simulink model "Red_problema6_rndm"  (R2021a)
settings: Solver=ode15s  StartTime=0.0  StopTime=sim_time  RelTol=1e-3
values from neighbouring files (symbols this model uses):
  aE112 = 177.25533427288616    (= 177.255334273)    [data_run_lazo_abierto_simulink.m]    (also in inicializar_areas.m = 179.376259805; script_IMC.m = a112_f)
  aE121 = 28.272251308900536    (= 28.2722513089)    [data_run_lazo_abierto_simulink.m]    (also in inicializar_areas.m; script_IMC.m = a121_f)
  aE213 = 304.960661680865    (= 304.960661681)    [data_run_lazo_abierto_simulink.m]    (also in inicializar_areas.m; script_IMC.m = a213_f)
  aE222 = 104.78323167686085    (= 104.783231677)    [data_run_lazo_abierto_simulink.m]    (also in inicializar_areas.m = 114.075570199; script_IMC.m = a222_f)
  aEcu1 = 2.44278466343862    (= 2.44278466344)    [data_run_lazo_abierto_simulink.m]    (also in inicializar_areas.m = 4.955447053)
  aEcu2 = 9.34130944614368    (= 9.34130944614)    [data_run_lazo_abierto_simulink.m]    (also in inicializar_areas.m = 18.78773145)
  aEhu2 = 53.1053199018638    (= 53.1053199019)    [data_run_lazo_abierto_simulink.m]    (also in inicializar_areas.m = 53.1053199)
  d1_end = 0    [data_run_lazo_abierto_simulink.m]    (also in inicializar_entradas.m; pert_max.m = 0.99; script_build_tfs.m)
  d1_in = 0    [data_run_lazo_abierto_simulink.m]    (also in inicializar_entradas.m; script_build_tfs.m)
  d2_end = 0    [data_run_lazo_abierto_simulink.m]    (also in inicializar_entradas.m; pert_max.m = 0.15; script_build_tfs.m)
  d2_in = 0    [data_run_lazo_abierto_simulink.m]    (also in inicializar_entradas.m; script_build_tfs.m)
  d3_end = 0    [data_run_lazo_abierto_simulink.m]    (also in inicializar_entradas.m; pert_max.m = 0.99; script_build_tfs.m)
  d3_in = 0    [data_run_lazo_abierto_simulink.m]    (also in inicializar_entradas.m; script_build_tfs.m)
  d4_end = 0    [data_run_lazo_abierto_simulink.m]    (also in inicializar_entradas.m; pert_max.m = 0.15; script_build_tfs.m)
  d4_in = 0    [data_run_lazo_abierto_simulink.m]    (also in inicializar_entradas.m; script_build_tfs.m)
  d5_end = 0    [data_run_lazo_abierto_simulink.m]    (also in inicializar_entradas.m; pert_max.m = -0.99; script_build_tfs.m)
  d5_in = 0    [data_run_lazo_abierto_simulink.m]    (also in inicializar_entradas.m; script_build_tfs.m)
  d6_end = 0    [data_run_lazo_abierto_simulink.m]    (also in inicializar_entradas.m; pert_max.m = 0.15; script_build_tfs.m)
  d6_in = 0    [data_run_lazo_abierto_simulink.m]    (also in inicializar_entradas.m; script_build_tfs.m)
  d7_end = 0    [data_run_lazo_abierto_simulink.m]    (also in inicializar_entradas.m; pert_max.m = -0.99; script_build_tfs.m)
  d7_in = 0    [data_run_lazo_abierto_simulink.m]    (also in inicializar_entradas.m; script_build_tfs.m)
  d8_end = 0    [data_run_lazo_abierto_simulink.m]    (also in inicializar_entradas.m; pert_max.m = 0.15; script_build_tfs.m)
  d8_in = 0    [data_run_lazo_abierto_simulink.m]    (also in inicializar_entradas.m; script_build_tfs.m)
  est = 1    [data_run_lazo_abierto_simulink.m]    (also in ini_comun.m; script_build_tfs.m)
  fc1 = 20    [data_run_lazo_abierto_simulink.m]    (also in ini_comun.m; script_build_tfs.m)
  fc2 = 50    [data_run_lazo_abierto_simulink.m]    (also in ini_comun.m; script_build_tfs.m)
  fcu1 = 36    [data_run_lazo_abierto_simulink.m]    (also in ini_comun.m = 1.45; inicializar_areas.m = 1.45; script_build_tfs.m = 1.45)
  fcu2 = 44    [data_run_lazo_abierto_simulink.m]    (also in ini_comun.m = 5; inicializar_areas.m = 5; script_build_tfs.m = 5)
  fh1 = 18    [data_run_lazo_abierto_simulink.m]    (also in ini_comun.m; script_build_tfs.m)
  fh2 = 22    [data_run_lazo_abierto_simulink.m]    (also in ini_comun.m; script_build_tfs.m)
  fhu2 = 14.8    [data_run_lazo_abierto_simulink.m]    (also in ini_comun.m = 15; inicializar_areas.m = 15; script_build_tfs.m = 15)
  hc1 = 1    [data_run_lazo_abierto_simulink.m]    (also in ini_comun.m; script_build_tfs.m)
  hc2 = 1    [data_run_lazo_abierto_simulink.m]    (also in ini_comun.m; script_build_tfs.m)
  hcu = 1    [data_run_lazo_abierto_simulink.m]    (also in ini_comun.m; script_build_tfs.m)
  hh1 = 1    [data_run_lazo_abierto_simulink.m]    (also in ini_comun.m; script_build_tfs.m)
  hh2 = 1    [data_run_lazo_abierto_simulink.m]    (also in ini_comun.m; script_build_tfs.m)
  hhu = 1    [data_run_lazo_abierto_simulink.m]    (also in ini_comun.m; script_build_tfs.m)
  nom_ini = initials    [data_run_lazo_abierto_simulink.m]    (also in script_build_tfs.m)
  s1 = 30    [data_run_lazo_abierto_simulink.m]    (also in ini_comun.m; script_build_tfs.m)
  salida_pto_op = [432.97111685 332.893814589 483.000816221 482.974592221]    [D_desc_v1.mat]    (also in D_full_v1.mat = [432.946215914 332.89088523 483.00068651 483.133358057]; D_spar_v1.mat = [432.948244916 332.889043395 483.001208597 483.133835705]; G_modelo_desc_v2.mat = [432.971365599 332.894094109 483.00091452 482.974592221]; G_modelo_desc_v3.mat = [432.971116863 332.893814604 483.000816226 482.974592221])
  t_step = 2000    [data_run_lazo_abierto_simulink.m]    (also in ini_comun.m = 20000; script_build_tfs.m = 1000)
  Tcin1 = 323    [data_run_lazo_abierto_simulink.m]    (also in ini_comun.m; script_build_tfs.m)
  Tcin2 = 433    [data_run_lazo_abierto_simulink.m]    (also in ini_comun.m; script_build_tfs.m)
  Tcuin = 288    [data_run_lazo_abierto_simulink.m]    (also in ini_comun.m; script_build_tfs.m)
  Thin1 = 543    [data_run_lazo_abierto_simulink.m]    (also in ini_comun.m; script_build_tfs.m)
  Thin2 = 493    [data_run_lazo_abierto_simulink.m]    (also in ini_comun.m; script_build_tfs.m)
  Thuin = 523    [data_run_lazo_abierto_simulink.m]    (also in ini_comun.m; script_build_tfs.m)
  u10_end = nom_ini(10)    [data_run_lazo_abierto_simulink.m]    (also in inicializar_entradas.m = initials(10); script_build_tfs.m)
  u10_in = nom_ini(10)    [data_run_lazo_abierto_simulink.m]    (also in inicializar_entradas.m = initials(10); script_build_tfs.m)
  u11_end = nom_ini(11)    [data_run_lazo_abierto_simulink.m]    (also in inicializar_entradas.m = initials(11); script_build_tfs.m)
  u11_in = nom_ini(11)    [data_run_lazo_abierto_simulink.m]    (also in inicializar_entradas.m = initials(11); script_build_tfs.m)
  u1_end = nom_ini(1)    [data_run_lazo_abierto_simulink.m]    (also in inicializar_entradas.m = initials(1); script_build_tfs.m)
  u1_in = nom_ini(1)    [data_run_lazo_abierto_simulink.m]    (also in inicializar_entradas.m = initials(1); script_build_tfs.m)
  u2_end = nom_ini(2)    [data_run_lazo_abierto_simulink.m]    (also in inicializar_entradas.m = initials(2); script_build_tfs.m)
  u2_in = nom_ini(2)    [data_run_lazo_abierto_simulink.m]    (also in inicializar_entradas.m = initials(2); script_build_tfs.m)
  u3_end = nom_ini(3)    [data_run_lazo_abierto_simulink.m]    (also in inicializar_entradas.m = initials(3); script_build_tfs.m)
  u3_in = nom_ini(3)    [data_run_lazo_abierto_simulink.m]    (also in inicializar_entradas.m = initials(3); script_build_tfs.m)
  u4_end = nom_ini(4)    [data_run_lazo_abierto_simulink.m]    (also in inicializar_entradas.m = initials(4); script_build_tfs.m)
  u4_in = nom_ini(4)    [data_run_lazo_abierto_simulink.m]    (also in inicializar_entradas.m = initials(4); script_build_tfs.m)
  u5_end = nom_ini(5)    [data_run_lazo_abierto_simulink.m]    (also in inicializar_entradas.m = initials(5); script_build_tfs.m)
  u5_in = nom_ini(5)    [data_run_lazo_abierto_simulink.m]    (also in inicializar_entradas.m = initials(5); script_build_tfs.m)
  u6_end = nom_ini(6)    [data_run_lazo_abierto_simulink.m]    (also in inicializar_entradas.m = initials(6); script_build_tfs.m)
  u6_in = nom_ini(6)    [data_run_lazo_abierto_simulink.m]    (also in inicializar_entradas.m = initials(6); script_build_tfs.m)
  u7_end = nom_ini(7)    [data_run_lazo_abierto_simulink.m]    (also in inicializar_entradas.m = initials(7); script_build_tfs.m)
  u7_in = nom_ini(7)    [data_run_lazo_abierto_simulink.m]    (also in inicializar_entradas.m = initials(7); script_build_tfs.m)
  u8_end = nom_ini(8)    [data_run_lazo_abierto_simulink.m]    (also in inicializar_entradas.m = initials(8); script_build_tfs.m)
  u8_in = nom_ini(8)    [data_run_lazo_abierto_simulink.m]    (also in inicializar_entradas.m = initials(8); script_build_tfs.m)
  u9_end = nom_ini(9)    [data_run_lazo_abierto_simulink.m]    (also in inicializar_entradas.m = initials(9); script_build_tfs.m)
  u9_in = nom_ini(9)    [data_run_lazo_abierto_simulink.m]    (also in inicializar_entradas.m = initials(9); script_build_tfs.m)
undefined symbols (not defined in the file or in its folder): amp_time, bypass_time, fail_constant, interval_time
libraries: simulink x34, cstblocks x1
(part 1 of 2)
settings Model: Creator=Lautaro  LastModifiedBy=fzpat
settings SolverCC: AlgebraicLoopSolver=TrustRegion
settings DataIOCC: InitialState=xFinal  LimitDataPoints=on  SaveFinalState=on  SaveFormat=Array  ReturnWorkspaceOutputs=off
settings OptimizationCC: BlockReduction=off  BooleanDataType=off  LifeSpan=inf
settings DebuggingCC: SaveWithParameterizedLinksMsg=none  UnderspecifiedInitializationDetection=Classic  MergeDetectMultiDrivingBlocksExec=none  SignalResolutionControl=TryResolveAllWithWarning  SFUnexpectedBacktrackingDiag=warning  SFNoUnconditionalDefaultTransitionDiag=warning  SFExecutionAtInitializationDiag=none  SFMachineParentedDataDiag=warning  ArithmeticOperatorsInVariantConditions=warning
settings HardwareCC: ProdBitPerPointer=32  ProdBitPerSizeT=32  ProdBitPerPtrDiffT=32  ProdLargestAtomicFloat=None  ProdIntDivRoundTo=Undefined  ProdEndianess=Unspecified  ProdWordSize=32  ProdHWDeviceType=32-bit Generic  TargetUnknown=on
settings ModelReferenceCC: PropagateSignalLabelsOutOfModel=off
settings SFSimCC: SimUseLocalCustomCode=off  CustomCodeUndefinedFunction=UseInterfaceOnly
settings RTWCC: RTWUseLocalCustomCode=off
settings CodeAppCC: StateflowObjectComments=on
settings GRTTargetCC: TargetLangStandard=C89/C90 (ANSI)
settings ConfigComp: CovMetricSettings=dw  CovSaveCumulativeToWorkspaceVar=on  CovSaveSingleToWorkspaceVar=on  CovExternalEMLEnable=off  CovSFcnEnable=off

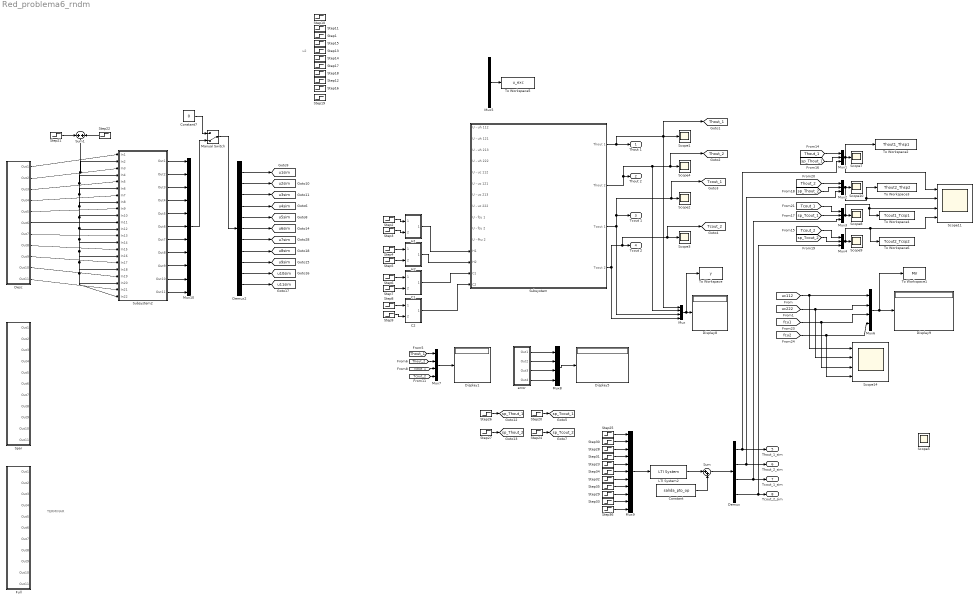
== system Red_problema6_rndm ==
  note: TERMINAR
  note: u2
  C1 : Subsystem
  "C2 " : Subsystem
  Constant : Constant  Value=salida_pto_op
  Constant7 : Constant  Value=0
  Demux : Demux
  Demux2 : Demux  Outputs=11
  Desc : Subsystem
  Display{1,5,8..9} (4 alike) : Display
  Full : Subsystem
  "H1 " : Subsystem
  H2 : Subsystem
  LTI System2 : cstblocks/LTI System  sys=G_modelo  IC=[]
  Manual Switch : ManualSwitch  CurrentSetting=0
  Mux{,6..8} (4 alike) : Mux
  Mux{1..4} (4 alike) : Mux  Inputs=3
  Mux10 : Mux  Inputs=11
  Mux5 : Mux  Inputs=11
  Mux9 : Mux  Inputs=11
  Scope{1..5,7..10} (9 alike) : Scope
  Scope11 : Scope  NumInputPorts=4
  Scope14 : Scope  NumInputPorts=4
  Spar : Subsystem
  Step1 : Step  Time=t_step  Before=u5_in  After=u5_end
  Step10 : Step  Time=t_step  Before=u1_in  After=u1_end
  Step11 : Step  Time=t_step  Before=u3_in  After=u3_end
  Step12 : Step  Time=t_step  Before=u9_in  After=u9_end
  Step13 : Step  Time=t_step  Before=u2_in  After=u2_end
  Step14 : Step  Time=t_step  Before=u4_in  After=u4_end
  Step15 : Step  Time=t_step  Before=u7_in  After=u7_end
  Step16 : Step  Time=t_step  Before=u10_in  After=u10_end
  Step17 : Step  Time=t_step  Before=u6_in  After=u6_end
  Step18 : Step  Time=t_step  Before=u8_in  After=u8_end
  Step19 : Step  Time=t_step  Before=u11_in  After=u11_end
  Step2 : Step  Time=t_step  Before=d1_in  After=d1_end
  Step20 : Step  Time=1e9  Before=210+273  After=210+273
  Step21 : Step  Time=bypass_time
  Step22 : Step  Time=bypass_time+125  After=-1
  Step23 : Step  Time=t_step  Before=u5_in - u5_in  After=u5_end - u5_in
  Step24 : Step  Time=1e10  Before=210+273  After=210+273
  Step25 : Step  Time=t_step  Before=u1_in - u1_in  After=u1_end - u1_in
  Step26 : Step  Time=1e9  Before=160+273  After=160+273
  Step27 : Step  Time=1e9  Before=60+273  After=60+273
  Step28 : Step  Time=t_step  Before=u3_in - u3_in  After=u3_end - u3_in
  Step29 : Step  Time=t_step  Before=u9_in - u9_in  After=u9_end - u9_in
  Step3 : Step  Time=t_step  Before=d2_in  After=d2_end
  Step30 : Step  Time=t_step  Before=u2_in - u2_in  After=u2_end - u2_in
  Step31 : Step  Time=t_step  Before=u4_in - u4_in  After=u4_end - u4_in
  Step32 : Step  Time=t_step  Before=u7_in - u7_in  After=u7_end - u7_in
  Step33 : Step  Time=t_step  Before=u10_in - u10_in  After=u10_end - u10_in
  Step34 : Step  Time=t_step  Before=u6_in - u6_in  After=u6_end - u6_in
  Step35 : Step  Time=t_step  Before=u8_in - u8_in  After=u8_end - u8_in
  Step36 : Step  Time=t_step  Before=u11_in - u11_in  After=u11_end - u11_in
  Step4 : Step  Time=t_step  Before=d3_in  After=d3_end
  Step5 : Step  Time=t_step  Before=d4_in  After=d4_end
  Step6 : Step  Time=t_step  Before=d5_in  After=d5_end
  Step7 : Step  Time=t_step  Before=d6_in  After=d6_end
  Step8 : Step  Time=t_step  Before=d7_in  After=d7_end
  Step9 : Step  Time=t_step  Before=d8_in  After=d8_end
  Subsystem : Subsystem
  Subsystem2 : Subsystem
  Sum : Sum  Inputs=|++
  Sum1 : Sum
  To Workspace : ToWorkspace  VariableName=y  SaveFormat=Timeseries  SampleTime=-1
  To Workspace1 : ToWorkspace  VariableName=MV  SaveFormat=Timeseries  SampleTime=-1
  To Workspace2 : ToWorkspace  VariableName=Thout1_Thsp1  SaveFormat=Timeseries  SampleTime=-1
  To Workspace3 : ToWorkspace  VariableName=Thout2_Thsp2  SampleTime=-1
  To Workspace4 : ToWorkspace  VariableName=Tcout1_Tcsp1  SampleTime=-1
  To Workspace5 : ToWorkspace  VariableName=u_exc  SaveFormat=Timeseries  SampleTime=-1
      settings: Save2DSignal=2-D array (concatenate along first dimension)
  To Workspace6 : ToWorkspace  VariableName=Tcout2_Tcsp2  SampleTime=-1
  error : Subsystem
  Thout 1 : Outport  VectorParamsAs1DForOutWhenUnconnected=off
  Thout 2 : Outport  Port=2  VectorParamsAs1DForOutWhenUnconnected=off
  Tcout 1 : Outport  Port=3  VectorParamsAs1DForOutWhenUnconnected=off
  Tcout 2 : Outport  Port=4  VectorParamsAs1DForOutWhenUnconnected=off
  Thout_1_sim : Outport  Port=5  VectorParamsAs1DForOutWhenUnconnected=off
  Thout_2_sim : Outport  Port=6  VectorParamsAs1DForOutWhenUnconnected=off
  Tcout_1_sim : Outport  Port=7  VectorParamsAs1DForOutWhenUnconnected=off
  Tcout_2_sim : Outport  Port=8  VectorParamsAs1DForOutWhenUnconnected=off
  tag scope: Tcout_1=global, Tcout_2=global, Thout_1=global, Thout_2=global, sp_Tcout_1=global, sp_Tcout_2=global, sp_Thout_1=global, sp_Thout_2=global, u10sim=global, u11sim=global, u1sim=global, u2sim=global, u3sim=global, u4sim=global, u5sim=global, u6sim=global, u7sim=global, u8sim=global, u9sim=global
  wires:
  Subsystem/1(Thout 1) -> Mux/1, Scope1/1, [Thout_1], Thout 1/1
  Mux/1 -> To Workspace/1, Display8/1
  "H1 "/1(Out1) -> Subsystem/12(H1)
  H2/1(Out1) -> Subsystem/13(H2)
  C1/1(Out1) -> Subsystem/14(C1)
  "C2 "/1(Out1) -> Subsystem/15(C2)
  Subsystem/2(Thout 2) -> [Thout_2], Scope4/1, Mux/2, Thout 2/1
  Subsystem/3(Tcout 1) -> [Tcout_1], Scope2/1, Tcout 1/1, Mux/3
  Step2/1 -> "H1 "/1(Thin 1)
  Step3/1 -> "H1 "/2(fhin 1)
  Step4/1 -> H2/1(Thin 2)
  Step5/1 -> H2/2(fhin 2)
  Step6/1 -> C1/1(Tcin 1)
  Step7/1 -> C1/2(fcin 1)
  Step8/1 -> "C2 "/1(Tcin 2)
  Step9/1 -> "C2 "/2(fcin 2)
  Subsystem/4(Tcout 2) -> [Tcout_2], Scope3/1, Tcout 2/1, Mux/4
  Mux7/1 -> Display1/1
  [Thout_1] -> Mux7/1
  [Thout_2] -> Mux7/2
  [Tcout_1] -> Mux7/3
  [Tcout_2] -> Mux7/4
  Mux8/1 -> Display5/1
  error/1(Out1) -> Mux8/1
  error/2(Out2) -> Mux8/2
  error/3(Out3) -> Mux8/3
  error/4(Out4) -> Mux8/4
  Mux6/1 -> To Workspace1/1, Display9/1
  [uc112] -> Mux6/1, Scope14/1
  [uc222] -> Mux6/2, Scope14/2
  [fcu1] -> Mux6/3, Scope14/3
  [fcu2] -> Scope14/4, Mux6/4
  Mux1/1 -> To Workspace2/1, Scope11/1, Scope7/1
  [sp_Thout_1] -> Mux1/2
  Mux2/1 -> To Workspace3/1, Scope11/2, Scope10/1
  [sp_Thout_2] -> Mux2/2
  Mux3/1 -> To Workspace4/1, Scope11/3, Scope8/1
  [sp_Tcout_1] -> Mux3/2
  Mux4/1 -> To Workspace6/1, Scope11/4, Scope9/1
  [sp_Tcout_2] -> Mux4/2
  [Thout_1] -> Mux1/1
  [Thout_2] -> Mux2/1
  [Tcout_1] -> Mux3/1
  [Tcout_2] -> Mux4/1
  Step20/1 -> [sp_Tcout_1]
  Step24/1 -> [sp_Tcout_2]
  Step26/1 -> [sp_Thout_1]
  Step27/1 -> [sp_Thout_2]
  Mux5/1 -> To Workspace5/1
  LTI System2/1 -> Sum/1
  Constant/1 -> Sum/2
  Mux9/1 -> LTI System2/1
  Sum/1 -> Demux/1
  Demux/1 -> Thout_1_sim/1, Mux1/3
  Demux/2 -> Mux2/3, Thout_2_sim/1
  Demux/3 -> Mux3/3, Tcout_1_sim/1
  Demux/4 -> Mux4/3, Tcout_2_sim/1
  Step25/1 -> Mux9/1
  Step30/1 -> Mux9/2
  Step28/1 -> Mux9/3
  Step31/1 -> Mux9/4
  Step23/1 -> Mux9/5
  Step34/1 -> Mux9/6
  Step32/1 -> Mux9/7
  Step35/1 -> Mux9/8
  Step29/1 -> Mux9/9
  Step33/1 -> Mux9/10
  Step36/1 -> Mux9/11
  Step22/1 -> Sum1/2
  Step21/1 -> Sum1/1
  Desc/1(Out1) -> Subsystem2/1(In1)
  Desc/2(Out2) -> Subsystem2/3(In3)
  Desc/3(Out3) -> Subsystem2/5(In5)
  Desc/4(Out4) -> Subsystem2/7(In7)
  Desc/5(Out5) -> Subsystem2/9(In9)
  Desc/7(Out7) -> Subsystem2/13(In13)
  Desc/6(Out6) -> Subsystem2/11(In11)
  Desc/8(Out8) -> Subsystem2/15(In15)
  Desc/9(Out9) -> Subsystem2/17(In17)
  Desc/10(Out10) -> Subsystem2/19(In19)
  Desc/11(Out11) -> Subsystem2/21(In21)
  Sum1/1 -> Subsystem2/22(In22), Subsystem2/20(In20), Subsystem2/18(In18), Subsystem2/16(In16), Subsystem2/14(In14), Subsystem2/12(In12), Subsystem2/10(In10), Subsystem2/8(In8), Subsystem2/6(In6), Subsystem2/4(In4), Subsystem2/2(In2)
  Manual Switch/1 -> Demux2/1
  Mux10/1 -> Manual Switch/2
  Constant7/1 -> Manual Switch/1
  Subsystem2/11(Out11) -> Mux10/11
  Subsystem2/10(Out10) -> Mux10/10
  Subsystem2/9(Out9) -> Mux10/9
  Subsystem2/8(Out8) -> Mux10/8
  Subsystem2/6(Out6) -> Mux10/6
  Subsystem2/5(Out5) -> Mux10/5
  Subsystem2/4(Out4) -> Mux10/4
  Subsystem2/3(Out3) -> Mux10/3
  Subsystem2/2(Out2) -> Mux10/2
  Subsystem2/1(Out1) -> Mux10/1
  Subsystem2/7(Out7) -> Mux10/7
  Demux2/1 -> [u1sim]
  Demux2/2 -> [u2sim]
  Demux2/3 -> [u3sim]
  Demux2/4 -> [u4sim]
  Demux2/5 -> [u5sim]
  Demux2/6 -> [u6sim]
  Demux2/7 -> [u7sim]
  Demux2/8 -> [u8sim]
  Demux2/9 -> [u9sim]
  Demux2/10 -> [u10sim]
  Demux2/11 -> [u11sim]

== system Red_problema6_rndm/C1 ==
  Tcin 1 : Inport
  fcin 1 : Inport  Port=2
  Add2 : Sum
  Add3 : Sum
  Constant3 : Constant  Value=Tcin1
  Constant4 : Constant  Value=fc1
  Mux5 : Mux  Inputs=3
  hc : Step  Before=hc1  After=hc1
  valvula : Subsystem
  Out1 : Outport  VectorParamsAs1DForOutWhenUnconnected=off
  wires:
  Constant3/1 -> Add2/1
  Constant4/1 -> Add3/1
  Tcin 1/1 -> Add2/2
  fcin 1/1 -> Add3/2
  Add2/1 -> Mux5/1
  Add3/1 -> Mux5/2
  hc/1 -> Mux5/3
  Mux5/1 -> valvula/1(In1)
  valvula/1(Out1) -> Out1/1

== system Red_problema6_rndm/C2  ==
  Tcin 2 : Inport
  fcin 2 : Inport  Port=2
  Add4 : Sum
  Add5 : Sum
  Constant5 : Constant  Value=Tcin2
  Constant6 : Constant  Value=fc2
  Mux5 : Mux  Inputs=3
  hc : Step  Before=hc2  After=hc2
  valvula : Subsystem
  Out1 : Outport  VectorParamsAs1DForOutWhenUnconnected=off
  wires:
  Constant5/1 -> Add4/1
  Constant6/1 -> Add5/1
  Tcin 2/1 -> Add4/2
  fcin 2/1 -> Add5/2
  Add4/1 -> Mux5/1
  Add5/1 -> Mux5/2
  hc/1 -> Mux5/3
  Mux5/1 -> valvula/1(In1)
  valvula/1(Out1) -> Out1/1

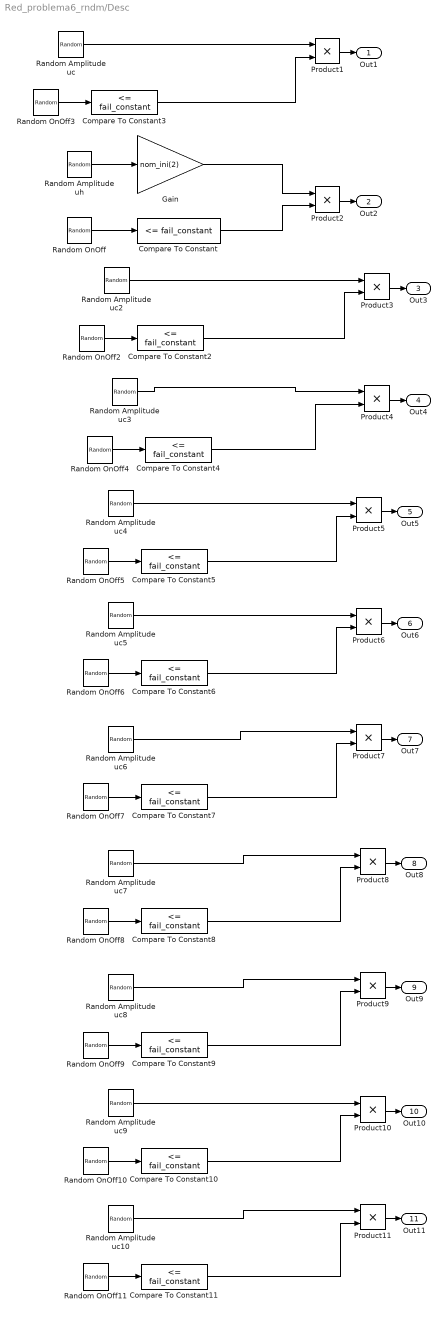
== system Red_problema6_rndm/Desc ==
  Compare To Constant{,2..11} (11 alike) : simulink/Logic and Bit Operations/Compare To Constant  relop=<=  const=fail_constant  OutDataTypeStr=boolean
  Gain : Gain  Gain=nom_ini(2)
  Product{1..11} (11 alike) : Product
  Random Amplitude uc : UniformRandomNumber  Minimum=0  Maximum=0.08  SampleTime=amp_time+3
  Random Amplitude uc10 : UniformRandomNumber  Minimum=0  Maximum=0.08  Seed=20  SampleTime=amp_time+3
  Random Amplitude uc2 : UniformRandomNumber  Minimum=0  Maximum=0.08  Seed=4  SampleTime=amp_time+3
  Random Amplitude uc3 : UniformRandomNumber  Minimum=0  Maximum=0.08  Seed=6  SampleTime=amp_time+3
  Random Amplitude uc4 : UniformRandomNumber  Minimum=0  Maximum=0.08  Seed=8  SampleTime=amp_time+3
  Random Amplitude uc5 : UniformRandomNumber  Minimum=0  Maximum=0.08  Seed=10  SampleTime=amp_time+3
  Random Amplitude uc6 : UniformRandomNumber  Minimum=0  Maximum=0.08  Seed=12  SampleTime=amp_time+3
  Random Amplitude uc7 : UniformRandomNumber  Minimum=0  Maximum=0.08  Seed=14  SampleTime=amp_time+3
  Random Amplitude uc8 : UniformRandomNumber  Minimum=0  Maximum=0.08  Seed=16  SampleTime=amp_time+3
  Random Amplitude uc9 : UniformRandomNumber  Minimum=0  Maximum=0.08  Seed=18  SampleTime=amp_time+3
  Random Amplitude uh : UniformRandomNumber  Minimum=-0.1  Maximum=0.1  SampleTime=amp_time+3
  Random OnOff : UniformRandomNumber  Minimum=0  Maximum=10  Seed=1  SampleTime=interval_time
  Random OnOff10 : UniformRandomNumber  Minimum=0  Maximum=10  Seed=19  SampleTime=interval_time
  Random OnOff11 : UniformRandomNumber  Minimum=0  Maximum=10  Seed=21  SampleTime=interval_time
  Random OnOff2 : UniformRandomNumber  Minimum=0  Maximum=10  Seed=5  SampleTime=interval_time
  Random OnOff3 : UniformRandomNumber  Minimum=0  Maximum=10  Seed=1  SampleTime=interval_time
  Random OnOff4 : UniformRandomNumber  Minimum=0  Maximum=10  Seed=7  SampleTime=interval_time
  Random OnOff5 : UniformRandomNumber  Minimum=0  Maximum=10  Seed=9  SampleTime=interval_time
  Random OnOff6 : UniformRandomNumber  Minimum=0  Maximum=10  Seed=11  SampleTime=interval_time
  Random OnOff7 : UniformRandomNumber  Minimum=0  Maximum=10  Seed=13  SampleTime=interval_time
  Random OnOff8 : UniformRandomNumber  Minimum=0  Maximum=10  Seed=15  SampleTime=interval_time
  Random OnOff9 : UniformRandomNumber  Minimum=0  Maximum=10  Seed=17  SampleTime=interval_time
  Out1 : Outport
  Out2 : Outport  Port=2
  Out3 : Outport  Port=3
  Out4 : Outport  Port=4
  Out5 : Outport  Port=5
  Out6 : Outport  Port=6
  Out7 : Outport  Port=7
  Out8 : Outport  Port=8
  Out9 : Outport  Port=9
  Out10 : Outport  Port=10
  Out11 : Outport  Port=11
  wires:
  Product1/1 -> Out1/1
  Random OnOff2/1 -> Compare To Constant2/1
  Random Amplitude uc3/1 -> Product4/1
  Compare To Constant7/1 -> Product7/2
  Random Amplitude uc7/1 -> Product8/1
  Random Amplitude uc8/1 -> Product9/1
  Compare To Constant9/1 -> Product9/2
  Compare To Constant8/1 -> Product8/2
  Random OnOff3/1 -> Compare To Constant3/1
  Random Amplitude uc2/1 -> Product3/1
  Random OnOff5/1 -> Compare To Constant5/1
  Random Amplitude uc5/1 -> Product6/1
  Product9/1 -> Out9/1
  Compare To Constant6/1 -> Product6/2
  Random Amplitude uc6/1 -> Product7/1
  Random Amplitude uh/1 -> Gain/1
  Compare To Constant10/1 -> Product10/2
  Random OnOff9/1 -> Compare To Constant9/1
  Compare To Constant4/1 -> Product4/2
  Compare To Constant11/1 -> Product11/2
  Random Amplitude uc9/1 -> Product10/1
  Product5/1 -> Out5/1
  Random OnOff/1 -> Compare To Constant/1
  Random OnOff4/1 -> Compare To Constant4/1
  Random Amplitude uc10/1 -> Product11/1
  Compare To Constant5/1 -> Product5/2
  Random OnOff10/1 -> Compare To Constant10/1
  Gain/1 -> Product2/1
  Random OnOff7/1 -> Compare To Constant7/1
  Random OnOff6/1 -> Compare To Constant6/1
  Product3/1 -> Out3/1
  Random Amplitude uc4/1 -> Product5/1
  Random Amplitude uc/1 -> Product1/1
  Product7/1 -> Out7/1
  Compare To Constant/1 -> Product2/2
  Product4/1 -> Out4/1
  Compare To Constant2/1 -> Product3/2
  Compare To Constant3/1 -> Product1/2
  Random OnOff11/1 -> Compare To Constant11/1
  Random OnOff8/1 -> Compare To Constant8/1
  Product6/1 -> Out6/1
  Product8/1 -> Out8/1
  Product2/1 -> Out2/1
  Product10/1 -> Out10/1
  Product11/1 -> Out11/1

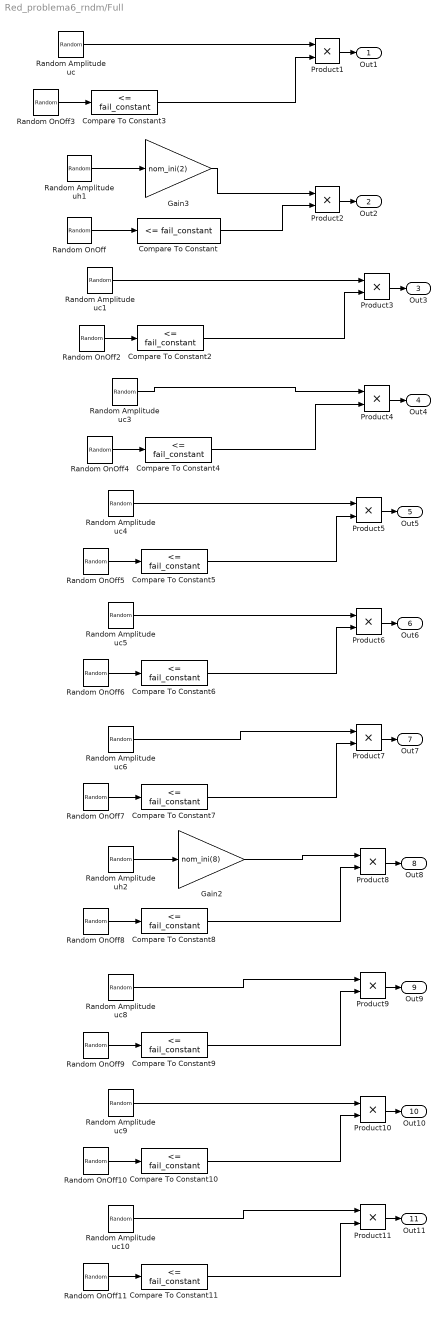
== system Red_problema6_rndm/Full ==
  Compare To Constant{,2..11} (11 alike) : simulink/Logic and Bit Operations/Compare To Constant  relop=<=  const=fail_constant  OutDataTypeStr=boolean
  Gain2 : Gain  Gain=nom_ini(8)
  Gain3 : Gain  Gain=nom_ini(2)
  Product{1..11} (11 alike) : Product
  Random Amplitude uc : UniformRandomNumber  Minimum=0  Maximum=0.08  SampleTime=amp_time+3
  Random Amplitude uc1 : UniformRandomNumber  Minimum=0  Maximum=0.08  Seed=2  SampleTime=amp_time+3
  Random Amplitude uc10 : UniformRandomNumber  Minimum=0  Maximum=0.08  Seed=20  SampleTime=amp_time+3
  Random Amplitude uc3 : UniformRandomNumber  Minimum=0  Maximum=0.08  Seed=6  SampleTime=amp_time+3
  Random Amplitude uc4 : UniformRandomNumber  Minimum=0  Maximum=0.08  Seed=8  SampleTime=amp_time+3
  Random Amplitude uc5 : UniformRandomNumber  Minimum=0  Maximum=0.08  Seed=10  SampleTime=amp_time+3
  Random Amplitude uc6 : UniformRandomNumber  Minimum=0  Maximum=0.08  Seed=12  SampleTime=amp_time+3
  Random Amplitude uc8 : UniformRandomNumber  Minimum=0  Maximum=0.08  Seed=16  SampleTime=amp_time+3
  Random Amplitude uc9 : UniformRandomNumber  Minimum=0  Maximum=0.08  Seed=18  SampleTime=amp_time+3
  Random Amplitude uh1 : UniformRandomNumber  Minimum=-0.1  Maximum=0.1  Seed=4  SampleTime=amp_time+3
  Random Amplitude uh2 : UniformRandomNumber  Minimum=-0.1  Maximum=0.1  Seed=14  SampleTime=amp_time+3
  Random OnOff : UniformRandomNumber  Minimum=0  Maximum=10  Seed=3  SampleTime=interval_time
  Random OnOff10 : UniformRandomNumber  Minimum=0  Maximum=10  Seed=19  SampleTime=interval_time
  Random OnOff11 : UniformRandomNumber  Minimum=0  Maximum=10  Seed=21  SampleTime=interval_time
  Random OnOff2 : UniformRandomNumber  Minimum=0  Maximum=10  Seed=5  SampleTime=interval_time
  Random OnOff3 : UniformRandomNumber  Minimum=0  Maximum=10  Seed=1  SampleTime=interval_time
  Random OnOff4 : UniformRandomNumber  Minimum=0  Maximum=10  Seed=7  SampleTime=interval_time
  Random OnOff5 : UniformRandomNumber  Minimum=0  Maximum=10  Seed=9  SampleTime=interval_time
  Random OnOff6 : UniformRandomNumber  Minimum=0  Maximum=10  Seed=11  SampleTime=interval_time
  Random OnOff7 : UniformRandomNumber  Minimum=0  Maximum=10  Seed=13  SampleTime=interval_time
  Random OnOff8 : UniformRandomNumber  Minimum=0  Maximum=10  Seed=15  SampleTime=interval_time
  Random OnOff9 : UniformRandomNumber  Minimum=0  Maximum=10  Seed=17  SampleTime=interval_time
  Out1 : Outport
  Out2 : Outport  Port=2
  Out3 : Outport  Port=3
  Out4 : Outport  Port=4
  Out5 : Outport  Port=5
  Out6 : Outport  Port=6
  Out7 : Outport  Port=7
  Out8 : Outport  Port=8
  Out9 : Outport  Port=9
  Out10 : Outport  Port=10
  Out11 : Outport  Port=11
  wires:
  Random Amplitude uh2/1 -> Gain2/1
  Gain2/1 -> Product8/1
  Product1/1 -> Out1/1
  Random OnOff2/1 -> Compare To Constant2/1
  Random Amplitude uc3/1 -> Product4/1
  Compare To Constant7/1 -> Product7/2
  Random Amplitude uc8/1 -> Product9/1
  Compare To Constant9/1 -> Product9/2
  Compare To Constant8/1 -> Product8/2
  Random OnOff3/1 -> Compare To Constant3/1
  Random OnOff5/1 -> Compare To Constant5/1
  Random Amplitude uc5/1 -> Product6/1
  Product9/1 -> Out9/1
  Compare To Constant6/1 -> Product6/2
  Random Amplitude uc6/1 -> Product7/1
  Compare To Constant10/1 -> Product10/2
  Random OnOff9/1 -> Compare To Constant9/1
  Compare To Constant4/1 -> Product4/2
  Compare To Constant11/1 -> Product11/2
  Random Amplitude uc9/1 -> Product10/1
  Product5/1 -> Out5/1
  Random OnOff/1 -> Compare To Constant/1
  Random OnOff4/1 -> Compare To Constant4/1
  Random Amplitude uc10/1 -> Product11/1
  Compare To Constant5/1 -> Product5/2
  Random OnOff10/1 -> Compare To Constant10/1
  Random OnOff7/1 -> Compare To Constant7/1
  Random OnOff6/1 -> Compare To Constant6/1
  Product3/1 -> Out3/1
  Random Amplitude uc4/1 -> Product5/1
  Random Amplitude uc/1 -> Product1/1
  Product7/1 -> Out7/1
  Compare To Constant/1 -> Product2/2
  Product4/1 -> Out4/1
  Compare To Constant2/1 -> Product3/2
  Compare To Constant3/1 -> Product1/2
  Random OnOff11/1 -> Compare To Constant11/1
  Random OnOff8/1 -> Compare To Constant8/1
  Product6/1 -> Out6/1
  Product8/1 -> Out8/1
  Product2/1 -> Out2/1
  Product10/1 -> Out10/1
  Product11/1 -> Out11/1
  Gain3/1 -> Product2/1
  Random Amplitude uh1/1 -> Gain3/1
  Random Amplitude uc1/1 -> Product3/1

== system Red_problema6_rndm/H1  ==
  Thin 1 : Inport
  fhin 1 : Inport  Port=2
  Add : Sum
  Add1 : Sum
  Constant1 : Constant  Value=Thin1
  Constant2 : Constant  Value=fh1
  Mux5 : Mux  Inputs=3
  hh : Step  Before=hh1  After=hh1
  valvula : Subsystem
  Out1 : Outport  VectorParamsAs1DForOutWhenUnconnected=off
  wires:
  Constant1/1 -> Add/1
  Thin 1/1 -> Add/2
  Add/1 -> Mux5/1
  Constant2/1 -> Add1/1
  fhin 1/1 -> Add1/2
  hh/1 -> Mux5/3
  Add1/1 -> Mux5/2
  Mux5/1 -> valvula/1(In1)
  valvula/1(Out1) -> Out1/1

== system Red_problema6_rndm/H2 ==
  Thin 2 : Inport
  fhin 2 : Inport  Port=2
  Add : Sum
  Add1 : Sum
  Constant1 : Constant  Value=Thin2
  Constant2 : Constant  Value=fh2
  Mux5 : Mux  Inputs=3
  hh : Step  Before=hh2  After=hh2
  valvula : Subsystem
  Out1 : Outport  VectorParamsAs1DForOutWhenUnconnected=off
  wires:
  Constant1/1 -> Add/1
  Thin 2/1 -> Add/2
  Add/1 -> Mux5/1
  Constant2/1 -> Add1/1
  fhin 2/1 -> Add1/2
  hh/1 -> Mux5/3
  Add1/1 -> Mux5/2
  Mux5/1 -> valvula/1(In1)
  valvula/1(Out1) -> Out1/1

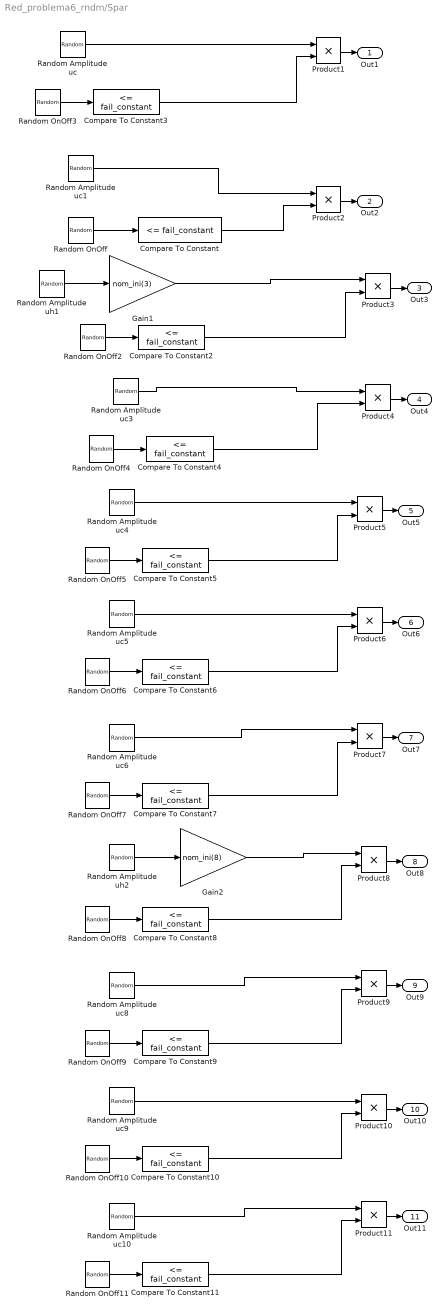
== system Red_problema6_rndm/Spar ==
  Compare To Constant{,2..11} (11 alike) : simulink/Logic and Bit Operations/Compare To Constant  relop=<=  const=fail_constant  OutDataTypeStr=boolean
  Gain1 : Gain  Gain=nom_ini(3)
  Gain2 : Gain  Gain=nom_ini(8)
  Product{1..11} (11 alike) : Product
  Random Amplitude uc : UniformRandomNumber  Minimum=0  Maximum=0.08  SampleTime=amp_time+3
  Random Amplitude uc1 : UniformRandomNumber  Minimum=0  Maximum=0.08  Seed=2  SampleTime=amp_time+3
  Random Amplitude uc10 : UniformRandomNumber  Minimum=0  Maximum=0.08  Seed=20  SampleTime=amp_time+3
  Random Amplitude uc3 : UniformRandomNumber  Minimum=0  Maximum=0.08  Seed=6  SampleTime=amp_time+3
  Random Amplitude uc4 : UniformRandomNumber  Minimum=0  Maximum=0.08  Seed=8  SampleTime=amp_time+3
  Random Amplitude uc5 : UniformRandomNumber  Minimum=0  Maximum=0.08  Seed=10  SampleTime=amp_time+3
  Random Amplitude uc6 : UniformRandomNumber  Minimum=0  Maximum=0.08  Seed=12  SampleTime=amp_time+3
  Random Amplitude uc8 : UniformRandomNumber  Minimum=0  Maximum=0.08  Seed=16  SampleTime=amp_time+3
  Random Amplitude uc9 : UniformRandomNumber  Minimum=0  Maximum=0.08  Seed=18  SampleTime=amp_time+3
  Random Amplitude uh1 : UniformRandomNumber  Minimum=-0.1  Maximum=0.1  Seed=4  SampleTime=amp_time+3
  Random Amplitude uh2 : UniformRandomNumber  Minimum=-0.1  Maximum=0.1  Seed=14  SampleTime=amp_time+3
  Random OnOff : UniformRandomNumber  Minimum=0  Maximum=10  Seed=3  SampleTime=interval_time
  Random OnOff10 : UniformRandomNumber  Minimum=0  Maximum=10  Seed=19  SampleTime=interval_time
  Random OnOff11 : UniformRandomNumber  Minimum=0  Maximum=10  Seed=21  SampleTime=interval_time
  Random OnOff2 : UniformRandomNumber  Minimum=0  Maximum=10  Seed=5  SampleTime=interval_time
  Random OnOff3 : UniformRandomNumber  Minimum=0  Maximum=10  Seed=1  SampleTime=interval_time
  Random OnOff4 : UniformRandomNumber  Minimum=0  Maximum=10  Seed=7  SampleTime=interval_time
  Random OnOff5 : UniformRandomNumber  Minimum=0  Maximum=10  Seed=9  SampleTime=interval_time
  Random OnOff6 : UniformRandomNumber  Minimum=0  Maximum=10  Seed=11  SampleTime=interval_time
  Random OnOff7 : UniformRandomNumber  Minimum=0  Maximum=10  Seed=13  SampleTime=interval_time
  Random OnOff8 : UniformRandomNumber  Minimum=0  Maximum=10  Seed=15  SampleTime=interval_time
  Random OnOff9 : UniformRandomNumber  Minimum=0  Maximum=10  Seed=17  SampleTime=interval_time
  Out1 : Outport
  Out2 : Outport  Port=2
  Out3 : Outport  Port=3
  Out4 : Outport  Port=4
  Out5 : Outport  Port=5
  Out6 : Outport  Port=6
  Out7 : Outport  Port=7
  Out8 : Outport  Port=8
  Out9 : Outport  Port=9
  Out10 : Outport  Port=10
  Out11 : Outport  Port=11
  wires:
  Product11/1 -> Out11/1
  Product10/1 -> Out10/1
  Product2/1 -> Out2/1
  Product8/1 -> Out8/1
  Product6/1 -> Out6/1
  Random OnOff8/1 -> Compare To Constant8/1
  Random OnOff11/1 -> Compare To Constant11/1
  Compare To Constant3/1 -> Product1/2
  Compare To Constant2/1 -> Product3/2
  Product4/1 -> Out4/1
  Compare To Constant/1 -> Product2/2
  Product7/1 -> Out7/1
  Random Amplitude uc/1 -> Product1/1
  Random Amplitude uc4/1 -> Product5/1
  Product3/1 -> Out3/1
  Random OnOff6/1 -> Compare To Constant6/1
  Random OnOff7/1 -> Compare To Constant7/1
  Random OnOff10/1 -> Compare To Constant10/1
  Compare To Constant5/1 -> Product5/2
  Random Amplitude uc10/1 -> Product11/1
  Random OnOff4/1 -> Compare To Constant4/1
  Random OnOff/1 -> Compare To Constant/1
  Product5/1 -> Out5/1
  Random Amplitude uc9/1 -> Product10/1
  Compare To Constant11/1 -> Product11/2
  Compare To Constant4/1 -> Product4/2
  Random OnOff9/1 -> Compare To Constant9/1
  Compare To Constant10/1 -> Product10/2
  Random Amplitude uc6/1 -> Product7/1
  Compare To Constant6/1 -> Product6/2
  Product9/1 -> Out9/1
  Random Amplitude uc5/1 -> Product6/1
  Random OnOff5/1 -> Compare To Constant5/1
  Random OnOff3/1 -> Compare To Constant3/1
  Compare To Constant8/1 -> Product8/2
  Compare To Constant9/1 -> Product9/2
  Random Amplitude uc8/1 -> Product9/1
  Compare To Constant7/1 -> Product7/2
  Random Amplitude uc3/1 -> Product4/1
  Random OnOff2/1 -> Compare To Constant2/1
  Product1/1 -> Out1/1
  Random Amplitude uh1/1 -> Gain1/1
  Gain1/1 -> Product3/1
  Gain2/1 -> Product8/1
  Random Amplitude uh2/1 -> Gain2/1
  Random Amplitude uc1/1 -> Product2/1

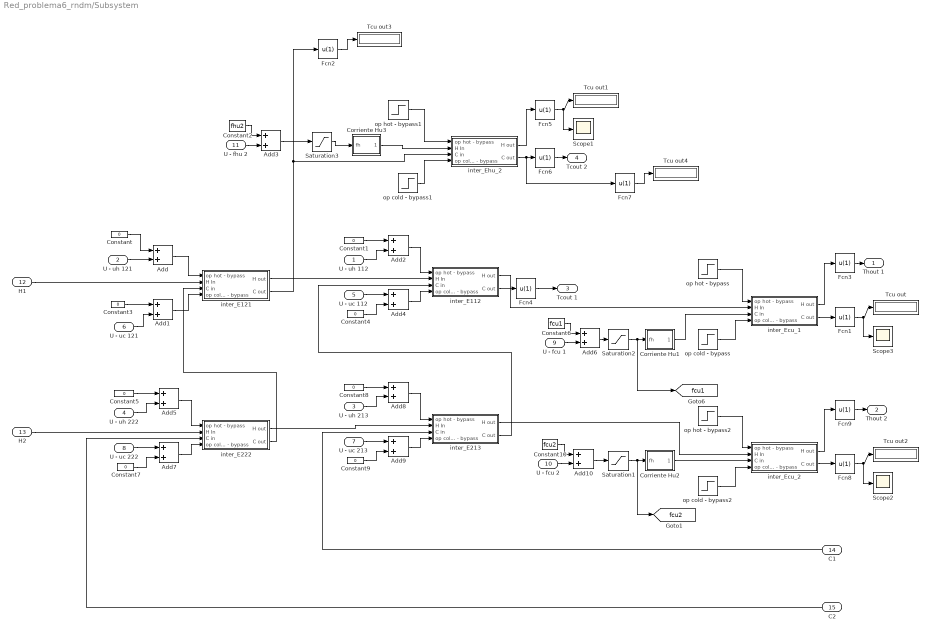
== system Red_problema6_rndm/Subsystem ==
  U - uh 112 : Inport
  U - uh 121 : Inport  Port=2
  U - uh 213 : Inport  Port=3
  U - uh 222 : Inport  Port=4
  U - uc 112 : Inport  Port=5
  U - uc 121 : Inport  Port=6
  U - uc 213 : Inport  Port=7
  U - uc 222 : Inport  Port=8
  U - fcu 1 : Inport  Port=9
  U - fcu 2 : Inport  Port=10
  U - fhu 2 : Inport  Port=11
  H1 : Inport  Port=12
  H2 : Inport  Port=13
  C1 : Inport  Port=14
  C2 : Inport  Port=15
  Add{,1..10} (11 alike) : Sum
  Constant{,1,3..5,7..9} (8 alike) : Constant  Value=0
  Constant10 : Constant  Value=fcu2
  Constant2 : Constant  Value=fhu2
  Constant6 : Constant  Value=fcu1
  Corriente Hu1 : Subsystem
  Corriente Hu2 : Subsystem
  Corriente Hu3 : Subsystem
  Fcn{1..9} (9 alike) : Fcn  Expr=u(1)
  Saturation1 : Saturate  UpperLimit=1e9  LowerLimit=0
  Saturation2 : Saturate  UpperLimit=1e9  LowerLimit=0
  Saturation3 : Saturate  UpperLimit=1e9  LowerLimit=0
  Scope1 : Scope
  Scope2 : Scope
  Scope3 : Scope
  Tcu out{,1..4} (5 alike) : Display
  inter_E112 : Subsystem
  inter_E121 : Subsystem
  inter_E213 : Subsystem
  inter_E222 : Subsystem
  inter_Ecu_1 : Subsystem
  inter_Ecu_2 : Subsystem
  inter_Ehu_2 : Subsystem
  op cold - bypass : Step  Time=0  After=0  SampleTime=0
  op cold - bypass1 : Step  Time=0  After=0  SampleTime=0
  op cold - bypass2 : Step  Time=0  After=0  SampleTime=0
  op hot - bypass : Step  Time=0  After=0  SampleTime=0
  op hot - bypass1 : Step  Time=0  After=0  SampleTime=0
  op hot - bypass2 : Step  Time=0  After=0  SampleTime=0
  Thout 1 : Outport  VectorParamsAs1DForOutWhenUnconnected=off
  Thout 2 : Outport  Port=2  VectorParamsAs1DForOutWhenUnconnected=off
  Tcout 1 : Outport  Port=3  VectorParamsAs1DForOutWhenUnconnected=off
  Tcout 2 : Outport  Port=4  VectorParamsAs1DForOutWhenUnconnected=off
  tag scope: fcu1=global, fcu2=global
  wires:
  op cold - bypass/1 -> inter_Ecu_1/4("op cold - bypass ")
  Fcn1/1 -> Scope3/1, Tcu out/1
  op hot - bypass/1 -> inter_Ecu_1/1("op hot - bypass ")
  U - uh 121/1 -> Add/2
  Constant/1 -> Add/1
  U - uc 121/1 -> Add1/2
  Add1/1 -> inter_E121/4("op cold - bypass ")
  Add/1 -> inter_E121/1("op hot - bypass ")
  U - uh 112/1 -> Add2/2
  Constant1/1 -> Add2/1
  Add2/1 -> inter_E112/1("op hot - bypass ")
  Constant3/1 -> Add1/1
  U - uc 112/1 -> Add4/1
  Constant4/1 -> Add4/2
  Add4/1 -> inter_E112/4("op cold - bypass ")
  Add6/1 -> Saturation2/1
  U - fcu 1/1 -> Add6/2
  Constant6/1 -> Add6/1
  op cold - bypass1/1 -> inter_Ehu_2/4("op cold - bypass ")
  Fcn5/1 -> Scope1/1, Tcu out1/1
  op hot - bypass1/1 -> inter_Ehu_2/1("op hot - bypass ")
  Add3/1 -> Saturation3/1
  U - fhu 2/1 -> Add3/2
  Constant2/1 -> Add3/1
  Corriente Hu3/1(Out1) -> inter_Ehu_2/2(H In)
  inter_Ehu_2/1(H out) -> Fcn5/1
  Fcn4/1 -> Tcout 1/1
  Fcn6/1 -> Tcout 2/1
  Fcn3/1 -> Thout 1/1
  inter_E121/1(H out) -> inter_E112/2(H In)
  Corriente Hu1/1(Out1) -> inter_Ecu_1/3(C in)
  inter_Ecu_1/2(C out) -> Fcn1/1
  inter_Ecu_1/1(H out) -> Fcn3/1
  U - uh 222/1 -> Add5/2
  Constant5/1 -> Add5/1
  Add5/1 -> inter_E222/1("op hot - bypass ")
  U - uc 222/1 -> Add7/1
  Constant7/1 -> Add7/2
  Add7/1 -> inter_E222/4("op cold - bypass ")
  U - uh 213/1 -> Add8/2
  Constant8/1 -> Add8/1
  Add8/1 -> inter_E213/1("op hot - bypass ")
  U - uc 213/1 -> Add9/1
  Constant9/1 -> Add9/2
  Add9/1 -> inter_E213/4("op cold - bypass ")
  H2/1 -> inter_E222/2(H In)
  inter_E222/1(H out) -> inter_E213/2(H In)
  op cold - bypass2/1 -> inter_Ecu_2/4("op cold - bypass ")
  Fcn8/1 -> Scope2/1, Tcu out2/1
  op hot - bypass2/1 -> inter_Ecu_2/1("op hot - bypass ")
  Add10/1 -> Saturation1/1
  U - fcu 2/1 -> Add10/2
  Constant10/1 -> Add10/1
  Fcn9/1 -> Thout 2/1
  Corriente Hu2/1(Out1) -> inter_Ecu_2/3(C in)
  inter_E213/1(H out) -> inter_Ecu_2/2(H In)
  inter_Ecu_2/2(C out) -> Fcn8/1
  inter_Ecu_2/1(H out) -> Fcn9/1
  C1/1 -> inter_E213/3(C in)
  C2/1 -> inter_E222/3(C in)
  inter_E121/2(C out) -> Fcn2/1, inter_Ehu_2/3(C in)
  Saturation3/1 -> Corriente Hu3/1(fh)
  Saturation2/1 -> [fcu1], Corriente Hu1/1(fh)
  Saturation1/1 -> [fcu2], Corriente Hu2/1(fh)
  Fcn2/1 -> Tcu out3/1
  inter_Ehu_2/2(C out) -> Fcn7/1, Fcn6/1
  Fcn7/1 -> Tcu out4/1
  H1/1 -> inter_E121/2(H In)
  inter_E222/2(C out) -> inter_E121/3(C in)
  inter_E112/1(H out) -> inter_Ecu_1/2(H In)
  inter_E112/2(C out) -> Fcn4/1
  inter_E213/2(C out) -> inter_E112/3(C in)

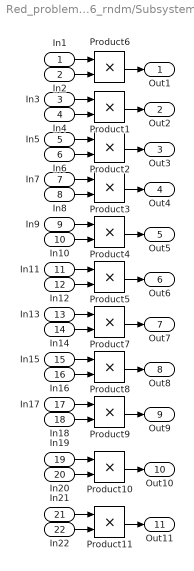
== system Red_problema6_rndm/Subsystem2 ==
  In1 : Inport
  In2 : Inport  Port=2
  In3 : Inport  Port=3
  In4 : Inport  Port=4
  In5 : Inport  Port=5
  In6 : Inport  Port=6
  In7 : Inport  Port=7
  In8 : Inport  Port=8
  In9 : Inport  Port=9
  In10 : Inport  Port=10
  In11 : Inport  Port=11
  In12 : Inport  Port=12
  In13 : Inport  Port=13
  In14 : Inport  Port=14
  In15 : Inport  Port=15
  In16 : Inport  Port=16
  In17 : Inport  Port=17
  In18 : Inport  Port=18
  In19 : Inport  Port=19
  In20 : Inport  Port=20
  In21 : Inport  Port=21
  In22 : Inport  Port=22
  Product{1..11} (11 alike) : Product
  Out1 : Outport
  Out2 : Outport  Port=2
  Out3 : Outport  Port=3
  Out4 : Outport  Port=4
  Out5 : Outport  Port=5
  Out6 : Outport  Port=6
  Out7 : Outport  Port=7
  Out8 : Outport  Port=8
  Out9 : Outport  Port=9
  Out10 : Outport  Port=10
  Out11 : Outport  Port=11
  wires:
  In11/1 -> Product5/1
  In6/1 -> Product2/2
  Product7/1 -> Out7/1
  Product11/1 -> Out11/1
  Product9/1 -> Out9/1
  Product2/1 -> Out3/1
  In9/1 -> Product4/1
  In2/1 -> Product6/2
  In8/1 -> Product3/2
  In10/1 -> Product4/2
  In5/1 -> Product2/1
  In18/1 -> Product9/2
  Product1/1 -> Out2/1
  In16/1 -> Product8/2
  Product4/1 -> Out5/1
  In15/1 -> Product8/1
  In19/1 -> Product10/1
  Product8/1 -> Out8/1
  In13/1 -> Product7/1
  Product5/1 -> Out6/1
  In7/1 -> Product3/1
  In17/1 -> Product9/1
  In12/1 -> Product5/2
  Product3/1 -> Out4/1
  In20/1 -> Product10/2
  Product10/1 -> Out10/1
  In14/1 -> Product7/2
  In21/1 -> Product11/1
  In22/1 -> Product11/2
  In3/1 -> Product1/1
  In1/1 -> Product6/1
  In4/1 -> Product1/2
  Product6/1 -> Out1/1

== system Red_problema6_rndm/error ==
  Add{,1..3} (4 alike) : Sum  Inputs=+-
  Out1 : Outport  VectorParamsAs1DForOutWhenUnconnected=off
  Out2 : Outport  Port=2  VectorParamsAs1DForOutWhenUnconnected=off
  Out3 : Outport  Port=3  VectorParamsAs1DForOutWhenUnconnected=off
  Out4 : Outport  Port=4  VectorParamsAs1DForOutWhenUnconnected=off
  wires:
  [sp_Thout_2] -> Add1/2
  [sp_Tcout_2] -> Add3/2
  [sp_Tcout_1] -> Add2/2
  [sp_Thout_1] -> Add/2
  [Thout_2] -> Add1/1
  [Thout_1] -> Add/1
  [Tcout_1] -> Add2/1
  [Tcout_2] -> Add3/1
  Add1/1 -> Out2/1
  Add/1 -> Out1/1
  Add3/1 -> Out4/1
  Add2/1 -> Out3/1

== system Red_problema6_rndm/C1/valvula ==
  In1 : Inport
  Gain : Gain  Gain=s1
  Gain1 : Gain  Gain=s1
  Integrator : Integrator  InitialCondition=[Tcin1 fc1 hc1]
  Sum : Sum  Inputs=|+-
  Out1 : Outport  VectorParamsAs1DForOutWhenUnconnected=off
  wires:
  Gain1/1 -> Sum/2
  Integrator/1 -> Gain1/1, Out1/1
  Sum/1 -> Integrator/1
  Gain/1 -> Sum/1
  In1/1 -> Gain/1

== system Red_problema6_rndm/C2 /valvula ==
  In1 : Inport
  Gain : Gain  Gain=s1
  Gain1 : Gain  Gain=s1
  Integrator : Integrator  InitialCondition=[Tcin2 fc2 hc2]
  Sum : Sum  Inputs=|+-
  Out1 : Outport  VectorParamsAs1DForOutWhenUnconnected=off
  wires:
  Gain1/1 -> Sum/2
  Integrator/1 -> Out1/1, Gain1/1
  Sum/1 -> Integrator/1
  Gain/1 -> Sum/1
  In1/1 -> Gain/1

== system Red_problema6_rndm/H1 /valvula ==
  In1 : Inport
  Gain : Gain  Gain=s1
  Gain1 : Gain  Gain=s1
  Integrator : Integrator  InitialCondition=[Thin1 fh1 hh1]
  Sum : Sum  Inputs=|+-
  Out1 : Outport  VectorParamsAs1DForOutWhenUnconnected=off
  wires:
  Gain1/1 -> Sum/2
  Integrator/1 -> Gain1/1, Out1/1
  Sum/1 -> Integrator/1
  Gain/1 -> Sum/1
  In1/1 -> Gain/1

== system Red_problema6_rndm/H2/valvula ==
  In1 : Inport
  Gain : Gain  Gain=s1
  Gain1 : Gain  Gain=s1
  Integrator : Integrator  InitialCondition=[Thin2 fh2 hh2]
  Sum : Sum  Inputs=|+-
  Out1 : Outport  VectorParamsAs1DForOutWhenUnconnected=off
  wires:
  Gain1/1 -> Sum/2
  Integrator/1 -> Gain1/1, Out1/1
  Sum/1 -> Integrator/1
  Gain/1 -> Sum/1
  In1/1 -> Gain/1

== system Red_problema6_rndm/Subsystem/Corriente Hu1 ==
  fh : Inport
  Mux5 : Mux  Inputs=3
  hh : Step  Before=1  SampleTime=0
  th : Step  Time=2  Before=15+273  After=15+273  SampleTime=0
  valvula 3 : Subsystem
  Out1 : Outport  VectorParamsAs1DForOutWhenUnconnected=off
  wires:
  hh/1 -> Mux5/3
  th/1 -> Mux5/1
  fh/1 -> Mux5/2
  Mux5/1 -> valvula 3/1(In1)
  valvula 3/1(Out1) -> Out1/1

== system Red_problema6_rndm/Subsystem/Corriente Hu2 ==
  fh : Inport
  Mux5 : Mux  Inputs=3
  hh : Step  Before=1  SampleTime=0
  th : Step  Time=2  Before=15+273  After=15+273  SampleTime=0
  valvula 3 : Subsystem
  Out1 : Outport  VectorParamsAs1DForOutWhenUnconnected=off
  wires:
  hh/1 -> Mux5/3
  th/1 -> Mux5/1
  fh/1 -> Mux5/2
  Mux5/1 -> valvula 3/1(In1)
  valvula 3/1(Out1) -> Out1/1

== system Red_problema6_rndm/Subsystem/Corriente Hu3 ==
  fh : Inport
  Mux5 : Mux  Inputs=3
  hh : Step  Before=1  SampleTime=0
  th : Step  Time=2  Before=250+273  After=250+273  SampleTime=0
  valvula 3 : Subsystem
  Out1 : Outport  VectorParamsAs1DForOutWhenUnconnected=off
  wires:
  hh/1 -> Mux5/3
  th/1 -> Mux5/1
  fh/1 -> Mux5/2
  Mux5/1 -> valvula 3/1(In1)
  valvula 3/1(Out1) -> Out1/1

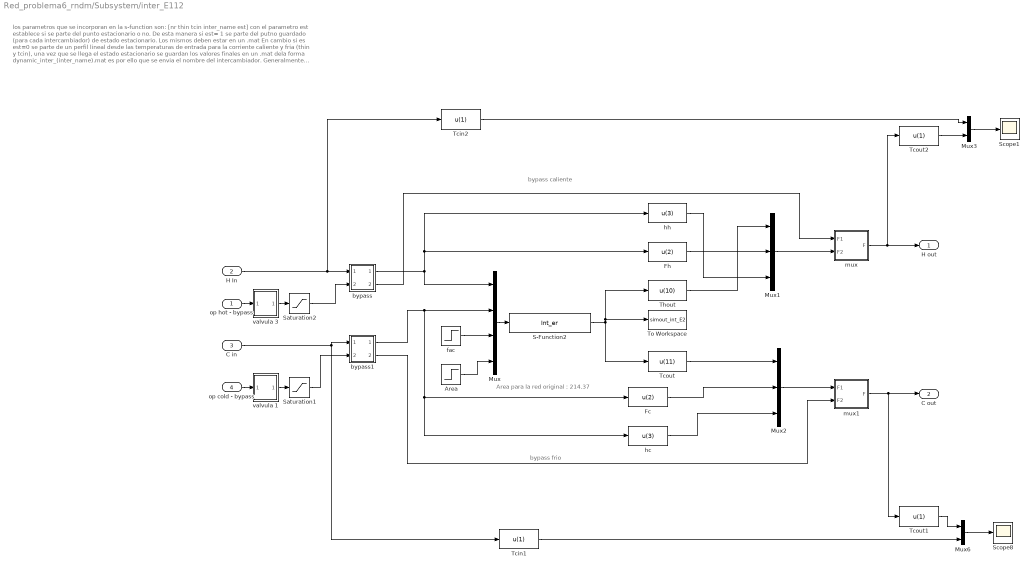
== system Red_problema6_rndm/Subsystem/inter_E112 ==
  note: Area para la red original : 214.37
  note: bypass caliente
  note: bypass frio
  note: los parametros que se incorporan en la s-function son: [nr thin tcin inter_name est]
      | con el parametro est establece si se parte del punto estacionario o no. De esta manera si est= 1 se parte del putno guardado (para cada intercambiador) de estado estacionario. Los mismos deben estar en un .mat
      | En cambio si es est=0 se parte de un perfil lineal  desde las temperaturas de entrada para la corriente caliente y fria (thin y tcin), una vez que se llega el estado estacionario se guardan los valores finales en un .mat
      | dela forma dynamic_inter_(inter_name).mat   es por ello que se envia el nombre del intercambiador.
      | Generalmente para la primera vez que se corre la red se una est=0 para que llegue al estado estacionario y una vez que se alcanzó se vuelve a correr con est= 1 para hacer análisis de control
  "op hot - bypass " : Inport
  H In : Inport  Port=2
  C in : Inport  Port=3
  "op cold - bypass " : Inport  Port=4
  Area : Step  Time=8  Before=aE112  After=aE112  SampleTime=0
  Fc : Fcn  Expr=u(2)
  Fh : Fcn  Expr=u(2)
  Mux : Mux
  Mux1 : Mux  Inputs=3
  Mux2 : Mux  Inputs=3
  Mux3 : Mux  Inputs=2
  Mux6 : Mux  Inputs=2
  S-Function2 : S-Function  FunctionName=Int_er  Parameters=10 528.5 433 112 est  SFunctionDeploymentMode=off  EnableBusSupport=off
  Saturation1 : Saturate  UpperLimit=1  LowerLimit=0
  Saturation2 : Saturate  UpperLimit=1  LowerLimit=0
  Scope1 : Scope
  Scope8 : Scope
  Tcin1 : Fcn  Expr=u(1)
  Tcin2 : Fcn  Expr=u(1)
  Tcout : Fcn  Expr=u(11)
  Tcout1 : Fcn  Expr=u(1)
  Tcout2 : Fcn  Expr=u(1)
  Thout : Fcn  Expr=u(10)
  To Workspace : ToWorkspace  VariableName=simout_int_E2  SampleTime=-1
  bypass : Subsystem
  bypass1 : Subsystem
  fac : Step  After=0  SampleTime=0
  hc : Fcn  Expr=u(3)
  hh : Fcn  Expr=u(3)
  mux : Subsystem
  mux1 : Subsystem
  valvula 1 : Subsystem
  valvula 3 : Subsystem
  H out : Outport  VectorParamsAs1DForOutWhenUnconnected=off
  C out : Outport  Port=2  VectorParamsAs1DForOutWhenUnconnected=off
  wires:
  Tcin2/1 -> Mux3/1
  Tcout2/1 -> Mux3/2
  Mux3/1 -> Scope1/1
  Tcin1/1 -> Mux6/2
  Tcout1/1 -> Mux6/1
  Mux6/1 -> Scope8/1
  bypass1/2(" 2") -> mux1/2(F2)
  bypass1/1(" 1") -> Mux/2, Fc/1, hc/1
  mux1/1("F ") -> C out/1, Tcout1/1
  Mux2/1 -> mux1/1(F1)
  mux/1("F ") -> H out/1, Tcout2/1
  C in/1 -> bypass1/1(1), Tcin1/1
  bypass/2(" 2") -> mux/1(F1)
  Mux1/1 -> mux/2(F2)
  bypass/1(" 1") -> hh/1, Fh/1, Mux/1
  H In/1 -> bypass/1(1), Tcin2/1
  Area/1 -> Mux/4
  hh/1 -> Mux1/3
  hc/1 -> Mux2/3
  fac/1 -> Mux/3
  Mux/1 -> S-Function2/1
  S-Function2/1 -> Tcout/1, To Workspace/1, Thout/1
  Fh/1 -> Mux1/2
  Fc/1 -> Mux2/2
  Thout/1 -> Mux1/1
  Tcout/1 -> Mux2/1
  Saturation1/1 -> bypass1/2(u122)
  Saturation2/1 -> bypass/2(u122)
  "op hot - bypass "/1 -> valvula 3/1(In1)
  "op cold - bypass "/1 -> valvula 1/1(In1)
  valvula 3/1(Out1) -> Saturation2/1
  valvula 1/1(Out1) -> Saturation1/1

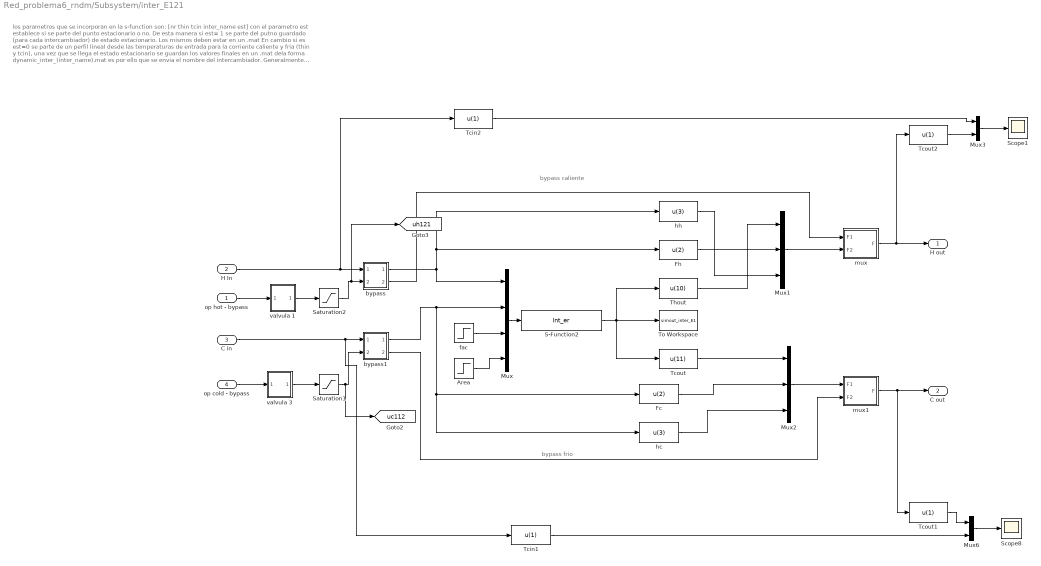
== system Red_problema6_rndm/Subsystem/inter_E121 ==
  note: los parametros que se incorporan en la s-function son: [nr thin tcin inter_name est]
      | con el parametro est establece si se parte del punto estacionario o no. De esta manera si est= 1 se parte del putno guardado (para cada intercambiador) de estado estacionario. Los mismos deben estar en un .mat
      | En cambio si es est=0 se parte de un perfil lineal  desde las temperaturas de entrada para la corriente caliente y fria (thin y tcin), una vez que se llega el estado estacionario se guardan los valores finales en un .mat
      | dela forma dynamic_inter_(inter_name).mat   es por ello que se envia el nombre del intercambiador.
      | Generalmente para la primera vez que se corre la red se una est=0 para que llegue al estado estacionario y una vez que se alcanzó se vuelve a correr con est= 1 para hacer análisis de control
  note: bypass frio
  note: bypass caliente
  "op hot - bypass " : Inport
  H In : Inport  Port=2
  C in : Inport  Port=3
  "op cold - bypass " : Inport  Port=4
  Area : Step  Time=0  Before=aE121  After=aE121  SampleTime=0
  Fc : Fcn  Expr=u(2)
  Fh : Fcn  Expr=u(2)
  Mux : Mux
  Mux1 : Mux  Inputs=3
  Mux2 : Mux  Inputs=3
  Mux3 : Mux  Inputs=2
  Mux6 : Mux  Inputs=2
  S-Function2 : S-Function  FunctionName=Int_er  Parameters=10 543 455 121 est  SFunctionDeploymentMode=off  EnableBusSupport=off
  Saturation1 : Saturate  UpperLimit=1  LowerLimit=0
  Saturation2 : Saturate  UpperLimit=1  LowerLimit=0
  Scope1 : Scope
  Scope8 : Scope
  Tcin1 : Fcn  Expr=u(1)
  Tcin2 : Fcn  Expr=u(1)
  Tcout : Fcn  Expr=u(11)
  Tcout1 : Fcn  Expr=u(1)
  Tcout2 : Fcn  Expr=u(1)
  Thout : Fcn  Expr=u(10)
  To Workspace : ToWorkspace  VariableName=simout_inter_E1  SampleTime=-1
  bypass : Subsystem
  bypass1 : Subsystem
  fac : Step  After=0  SampleTime=0
  hc : Fcn  Expr=u(3)
  hh : Fcn  Expr=u(3)
  mux : Subsystem
  mux1 : Subsystem
  valvula 1 : Subsystem
  valvula 3 : Subsystem
  H out : Outport  VectorParamsAs1DForOutWhenUnconnected=off
  C out : Outport  Port=2  VectorParamsAs1DForOutWhenUnconnected=off
  tag scope: uc112=global, uh121=global
  wires:
  Tcout/1 -> Mux2/1
  Thout/1 -> Mux1/1
  Fc/1 -> Mux2/2
  Fh/1 -> Mux1/2
  S-Function2/1 -> Thout/1, To Workspace/1, Tcout/1
  Mux/1 -> S-Function2/1
  fac/1 -> Mux/3
  hc/1 -> Mux2/3
  hh/1 -> Mux1/3
  Area/1 -> Mux/4
  H In/1 -> Tcin2/1, bypass/1(1)
  bypass/1(" 1") -> Mux/1, Fh/1, hh/1
  Mux1/1 -> mux/2(F2)
  bypass/2(" 2") -> mux/1(F1)
  C in/1 -> Tcin1/1, bypass1/1(1)
  mux/1("F ") -> Tcout2/1, H out/1
  Mux2/1 -> mux1/1(F1)
  mux1/1("F ") -> Tcout1/1, C out/1
  bypass1/1(" 1") -> hc/1, Fc/1, Mux/2
  bypass1/2(" 2") -> mux1/2(F2)
  Mux6/1 -> Scope8/1
  Tcout1/1 -> Mux6/1
  Tcin1/1 -> Mux6/2
  Mux3/1 -> Scope1/1
  Tcout2/1 -> Mux3/2
  Tcin2/1 -> Mux3/1
  Saturation1/1 -> [uc112], bypass1/2(u122)
  Saturation2/1 -> [uh121], bypass/2(u122)
  "op cold - bypass "/1 -> valvula 3/1(In1)
  "op hot - bypass "/1 -> valvula 1/1(In1)
  valvula 3/1(Out1) -> Saturation1/1
  valvula 1/1(Out1) -> Saturation2/1
